simulink model "Dynamic_velocity"  (R2019a)
settings: Solver=ode3  StartTime=0.0  StopTime=40  FixedStep=0.005  RelTol=1e-3
settings Model: Creator=ADMIN  LastModifiedBy=ADMIN

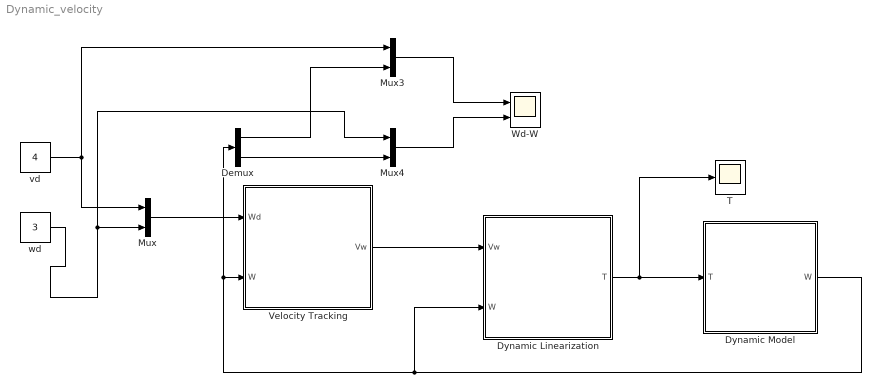
== system Dynamic_velocity ==
  Demux : Demux  Outputs=2
  Dynamic Linearization : Subsystem
  Dynamic Model : Subsystem  mask{v0=-4, w0=0}
      mask TypeOptions v0: v0/InitialCondition
      mask TypeOptions w0: w0/InitialCondition
  Mux : Mux  Inputs=2
  Mux3 : Mux  Inputs=2
  Mux4 : Mux  Inputs=2
  T : Scope
  Velocity Tracking : Subsystem  mask{Kv=[6; 0.6]}
      mask TypeOptions Kv: Kv/Gain
  Wd-W : Scope  NumInputPorts=2
  vd : Constant  Value=4
  wd : Constant  Value=3
  wires:
  Dynamic Linearization/1(T) -> T/1, Dynamic Model/1(T)
  Velocity Tracking/1(Vw) -> Dynamic Linearization/1(Vw)
  vd/1 -> Mux/1, Mux3/1
  Mux/1 -> Velocity Tracking/1(Wd)
  Mux4/1 -> Wd-W/2
  Dynamic Model/1(W) -> Demux/1, Velocity Tracking/2(W), Dynamic Linearization/2(W)
  Mux3/1 -> Wd-W/1
  Demux/2 -> Mux4/2
  Demux/1 -> Mux3/2
  wd/1 -> Mux4/1, Mux/2

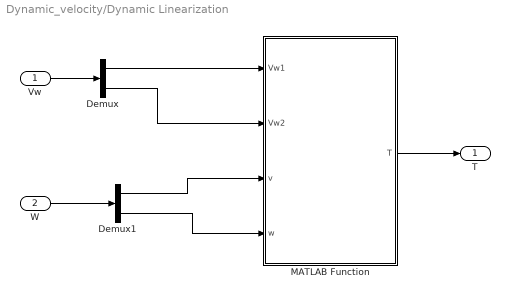
== system Dynamic_velocity/Dynamic Linearization ==
  Vw : Inport
  W : Inport  Port=2
  Demux : Demux  Outputs=2
  Demux1 : Demux  Outputs=2
  MATLAB Function : MATLAB Function  TreatAsAtomicUnit=on
  T : Outport
  wires:
  MATLAB Function/1(T) -> T/1
  Vw/1 -> Demux/1
  Demux/1 -> MATLAB Function/1(Vw1)
  Demux/2 -> MATLAB Function/2(Vw2)
  W/1 -> Demux1/1
  Demux1/1 -> MATLAB Function/3(v)
  Demux1/2 -> MATLAB Function/4(w)

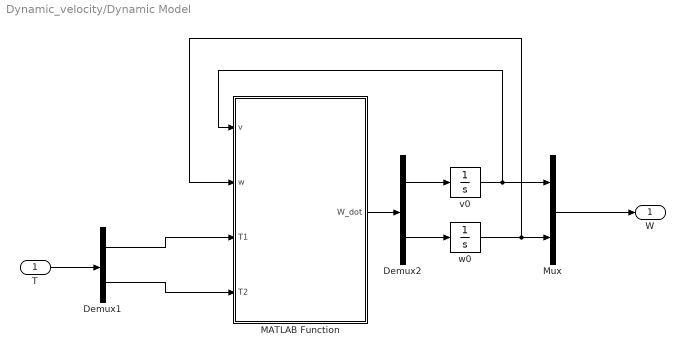
== system Dynamic_velocity/Dynamic Model ==
  T : Inport
  Demux1 : Demux  Outputs=2
  Demux2 : Demux  Outputs=2
  MATLAB Function : MATLAB Function  TreatAsAtomicUnit=on
  Mux : Mux  Inputs=2
  v0 : Integrator  InitialCondition=v0
  w0 : Integrator  InitialCondition=w0
  W : Outport
  wires:
  MATLAB Function/1(W_dot) -> Demux2/1
  Demux2/2 -> w0/1
  Demux2/1 -> v0/1
  v0/1 -> MATLAB Function/1(v), Mux/1
  w0/1 -> MATLAB Function/2(w), Mux/2
  Mux/1 -> W/1
  T/1 -> Demux1/1
  Demux1/1 -> MATLAB Function/3(T1)
  Demux1/2 -> MATLAB Function/4(T2)

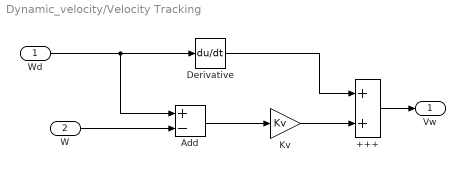
== system Dynamic_velocity/Velocity Tracking ==
  Wd : Inport
  W : Inport  Port=2
  +++ : Sum
  Add : Sum  Inputs=+-
  Derivative : Derivative
  Kv : Gain  Gain=Kv
  Vw : Outport
  wires:
  +++/1 -> Vw/1
  Derivative/1 -> +++/1
  Kv/1 -> +++/2
  Add/1 -> Kv/1
  W/1 -> Add/2
  Wd/1 -> Add/1, Derivative/1

== matlab function Dynamic_velocity/Dynamic Model/MATLAB Function ==
  data: v input; w input; T1 input; T2 input; W_dot output
function W_dot = fcn(v,w,T1,T2)
%% Parameters
r = 0.05;   %% (m) bán kính bánh xe
L = 0.27/2; %% L (m): khoang cach tu banh xe den truc
m = 4;      %% (kg) Mass of robot
I = 2.5;    %% (kg.m^2) Moment of inertia of whole robot
d = 0.05;   %% (m) Distance from point p0 to point pc
a = r/2;
b = r/(2*L);
%%
M_ = [m*a^2 + I*b^2, m*a^2 - I*b^2;
      m*a^2 - I*b^2, m*a^2 + I*b^2];

C_ = [0,        -2*a*b*d*m*w;
      2*a*b*d*m*w,  0];
B_ = [1,0;0,1];
%%
T = [T1;T2];
W = [v;w];
%%
W_dot = -inv(M_)*C_*W + inv(M_)*B_*T;
end

== matlab function Dynamic_velocity/Dynamic Linearization/MATLAB Function ==
  data: Vw1 input; Vw2 input; v input; w input; T output
function T = fcn(Vw1,Vw2,v,w)
%% Parameters
r = 0.05;   %% (m) bán kính bánh xe
L = 0.27/2; %% L (m): khoang cach tu banh xe den truc
m = 4;      %% (kg) Mass of robot
I = 2.5;    %% (kg.m^2) Moment of inertia of whole robot
d = 0.05;   %% (m) Distance from point p0 to point pc
a= r/2;
b = r/(2*L);
%%
M_ = [m*a^2 + I*b^2, m*a^2 - I*b^2;
      m*a^2 - I*b^2, m*a^2 + I*b^2];

C_ = [0,        -2*a*b*d*m*w;
      2*a*b*d*m*w,  0];
B_ = [1,0;0,1];
%%
Vw = [Vw1;Vw2];
W = [v;w];
%%
T = inv(B_)*M_*(Vw + inv(M_)*C_*W);
end
